simulink model "VectorCtrl_Asynchronous_VF"  (Simulink 7.9)
settings: Solver=ode23tb  StartTime=0.0  StopTime=6  RelTol=1e-3
InitFcn:
  | np=2;
  | Ts=50e-6;
  | fbase=50;
  | Vbase=440*sqrt(2/3);
libraries: powerlib x6, simulink x4, powerlib_extras x1
settings Model: Creator=H002220  LastModifiedBy=H002220

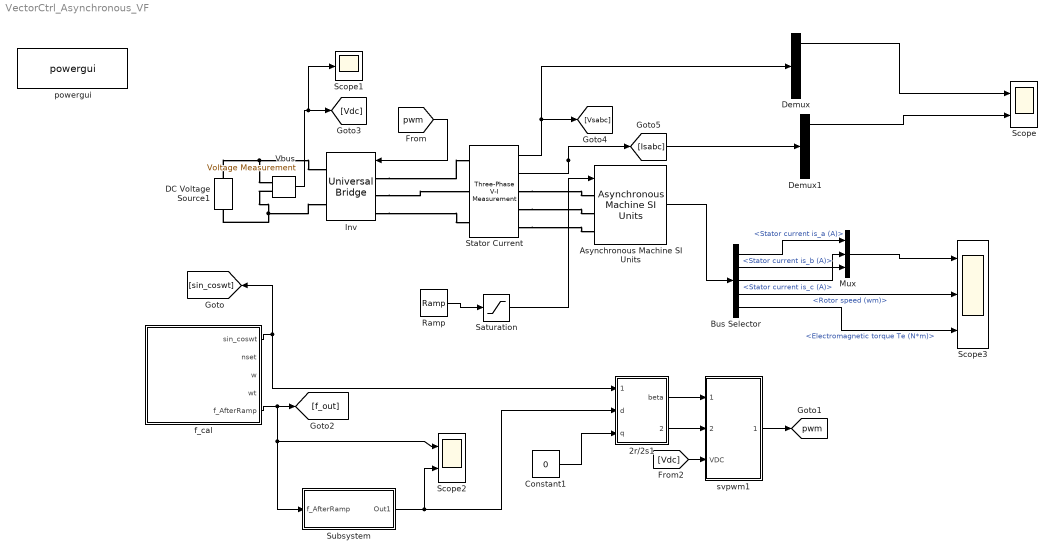
== system VectorCtrl_Asynchronous_VF ==
  2r/2s1 : Subsystem
  Asynchronous Machine SI Units : powerlib/Machines/Asynchronous Machine SI Units  PresetModel="18:  50 HP (37KW)   400 V 50Hz 1480 RPM"  MechanicalLoad=Torque Tm  ShowDetailedParameters=on  RotorType=Squirrel-cage  ReferenceFrame=Rotor  NominalParameters=[3.7e+04 400 50]  Stator=[0.08233 0.000724]  Rotor=[0.0503 0.000724]  Cage1=[ 0.022 0.226/377]  Cage2=[ 0.022 0.226/377]  Lm=0.02711  Mechanical=[0.37 0.02791 2]  PolePairs=2  InitialConditions=[1 0 0 0 0 0 0 0]  Units=SI  LoadFlowParameters=1492000  SimulateSaturation=off  Saturation=[14.03593122, 27.81365428, 53.79336849, 72.68890987, 97.98006896, 148.6815601, 215.7428561, 302.9841135, 420.4778367 ; 230, 322, 414, 460, 506, 552, 598, 644, 690]  TsPowergui=0  TsBlock=-1  IterativeModel=Forward Euler  Pmec=0
  Bus Selector : BusSelector  OutputSignals=Stator measurements.Stator current is_a (A),Stator measurements.Stator current is_b (A),Stator measurements.Stator current is_c (A),Mechanical.Rotor speed (wm),Mechanical.Electromagnetic torque Te (N*m)
  Constant1 : Constant  Value=0
  DC Voltage Source1 : powerlib/Electrical Sources/DC Voltage Source  Amplitude=600  Measurements=None
  Demux : Demux  Outputs=3
  Demux1 : Demux  Outputs=3
  Inv : powerlib/Power Electronics/Universal Bridge  Arms=3  SnubberResistance=1e5  SnubberCapacitance=inf  Device=IGBT / Diodes  Ron=1e-3  Lon=0  ForwardVoltages="[  0  0  ]"  ForwardVoltage=0  GTOparameters=[ 10e-6 , 20e-6 ]  IGBTparameters=[ 1e-6 , 2e-6 ]  Measurements=None  Measurements_2=None  converterType=Rectifier
  Mux : Mux  Inputs=3
  Ramp : simulink/Sources/Ramp  slope=4  start=0  X0=0
  Saturation : Saturate  UpperLimit=20  LowerLimit=0
  Scope : Scope  NumInputPorts=2
      settings: YMin=-5~-5  YMax=5~5  SaveName=a
  Scope1 : Scope
      settings: SaveName=ScopeData3
  Scope2 : Scope  NumInputPorts=2
      settings: YMin=-5~-5  YMax=5~5  SaveName=ScopeData4
  Scope3 : Scope  NumInputPorts=3
      settings: YMin=-5~-5~-5  YMax=5~5~5  SaveName=ScopeData5
  Stator Current : powerlib/Measurements/Three-Phase V-I Measurement  VoltageMeasurement=phase-to-phase  SetLabelV=off  LabelV=Vabc  Vpu=off  VpuLL=off  CurrentMeasurement=yes  SetLabelI=off  LabelI=Iabc  Ipu=off  Pbase=100e6  Vbase=500e3  OutputType=Complex  PhasorSimulation=off  PSBequivalent=0
  Subsystem : Subsystem
  Vbus : powerlib/Measurements/Voltage Measurement  PhasorSimulation=off  OutputType=Complex  PSBequivalent=0
  f_cal : Subsystem
  powergui : powerlib/powergui  SimulationMode=Discrete  SolverType=Tustin  SampleTime=50e-6  frequency=60  SPID=off  DisableSnubberDevices=off  DisableRonSwitches=off  DisableVfSwitches=off  SwTol=0  Interpol=off  DisplayEquations=off  FunctionMessages=off  frequencyindice=0  Pbase=100e6  ErrMax=1e-4  Iterations=50  UnitsV=kV  UnitsW=MW  echomessages=off  HookPort=off  EnableUseOfTLC=off  x0status=blocks  RestoreLinks=warning  ResistiveCurrentMeasurement=off  Frange=[0:2:500]  Ylog=off  Xlog=on  ShowGrid=off  save=off  variable=ZData  structure=a  ZoomFFT=off  StartTime=4.5  cycles=10  DisplayStyle=2  fundamental=45  FreqAxis=on  MaxFrequency=1000  frequencyindicesteady=1  RmsSteady=1  display=off  Ts=0  methode=off
  svpwm1 : Subsystem
  tag scope: pwm=global
  wires:
  2r/2s1/2(alpha) -> svpwm1/2(usaref)
  2r/2s1/1(beta) -> svpwm1/1(usbref)
  svpwm1/1(6pulse) -> [pwm]
  [Vdc] -> svpwm1/3(VDC)
  Subsystem/1(Out1) -> 2r/2s1/2(d), Scope2/2
  Constant1/1 -> 2r/2s1/3(q)
  Vbus/1 -> [Vdc], Scope1/1
  Stator Current/1 -> [Vsabc], Demux/1
  Stator Current/2 -> [Isabc], Demux1/1
  [pwm] -> Inv/1
  f_cal/5(f_AfterRamp) -> [f_out], Subsystem/1(f_AfterRamp), Scope2/1
  f_cal/1(sin_coswt) -> [sin_coswt], 2r/2s1/1(sin_cos)
  Demux/1 -> Scope/1
  Demux1/1 -> Scope/2
  Asynchronous Machine SI Units/1 -> Bus Selector/1
  Ramp/1 -> Saturation/1
  Saturation/1 -> Asynchronous Machine SI Units/1
  Bus Selector/1 -> Mux/1  "<Stator current is_a (A)>"
  Bus Selector/2 -> Mux/2  "<Stator current is_b (A)>"
  Bus Selector/3 -> Mux/3  "<Stator current is_c (A)>"
  Mux/1 -> Scope3/1
  Bus Selector/4 -> Scope3/2  "<Rotor speed (wm)>"
  Bus Selector/5 -> Scope3/3  "<Electromagnetic torque Te (N*m)>"
  connections:
  Inv/LConn1 -- Stator Current/LConn1
  Inv/LConn2 -- Stator Current/LConn2
  Inv/LConn3 -- Stator Current/LConn3
  Vbus/LConn2 -- Inv/RConn2 -- DC Voltage Source1/LConn1
  Stator Current/RConn3 -- Asynchronous Machine SI Units/LConn3
  Stator Current/RConn2 -- Asynchronous Machine SI Units/LConn2
  Stator Current/RConn1 -- Asynchronous Machine SI Units/LConn1
  DC Voltage Source1/RConn1 -- Inv/RConn1 -- Vbus/LConn1

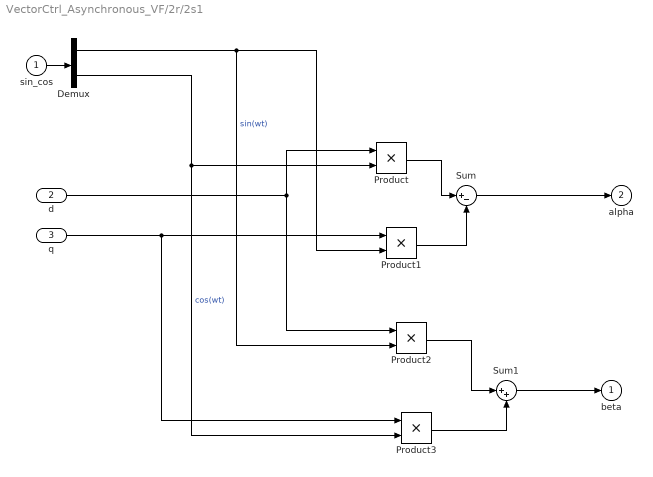
== system VectorCtrl_Asynchronous_VF/2r/2s1 ==
  sin_cos : Inport  PortDimensions=2
  d : Inport  Port=2
  q : Inport  Port=3
  Demux : Demux  Outputs=2
  Product{,1..3} (4 alike) : Product  RndMeth=Zero
  Sum : Sum  Inputs=|+-
  Sum1 : Sum  Inputs=|++
  beta : Outport  InitialOutput=0
  alpha : Outport  Port=2  InitialOutput=0
  wires:
  Sum/1 -> alpha/1
  Demux/1 -> Product1/2, Product2/2  "sin(wt)"
  Demux/2 -> Product/2, Product3/2  "cos(wt)"
  sin_cos/1 -> Demux/1
  d/1 -> Product/1, Product2/1
  q/1 -> Product1/1, Product3/1
  Product/1 -> Sum/1
  Product1/1 -> Sum/2
  Product2/1 -> Sum1/1
  Product3/1 -> Sum1/2
  Sum1/1 -> beta/1

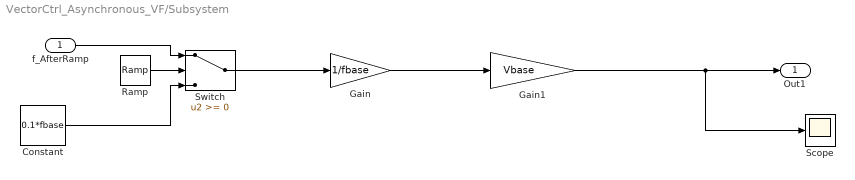
== system VectorCtrl_Asynchronous_VF/Subsystem ==
  f_AfterRamp : Inport
  Constant : Constant  Value=0.1*fbase
  Gain : Gain  Gain=1/fbase
  Gain1 : Gain  Gain=Vbase
  Ramp : simulink/Sources/Ramp  slope=1  start=0  X0=0
  Scope : Scope
      settings: SaveName=ScopeData6
  Switch : Switch
  Out1 : Outport
  wires:
  Gain/1 -> Gain1/1
  Gain1/1 -> Out1/1, Scope/1
  Ramp/1 -> Switch/2
  f_AfterRamp/1 -> Switch/1
  Constant/1 -> Switch/3
  Switch/1 -> Gain/1

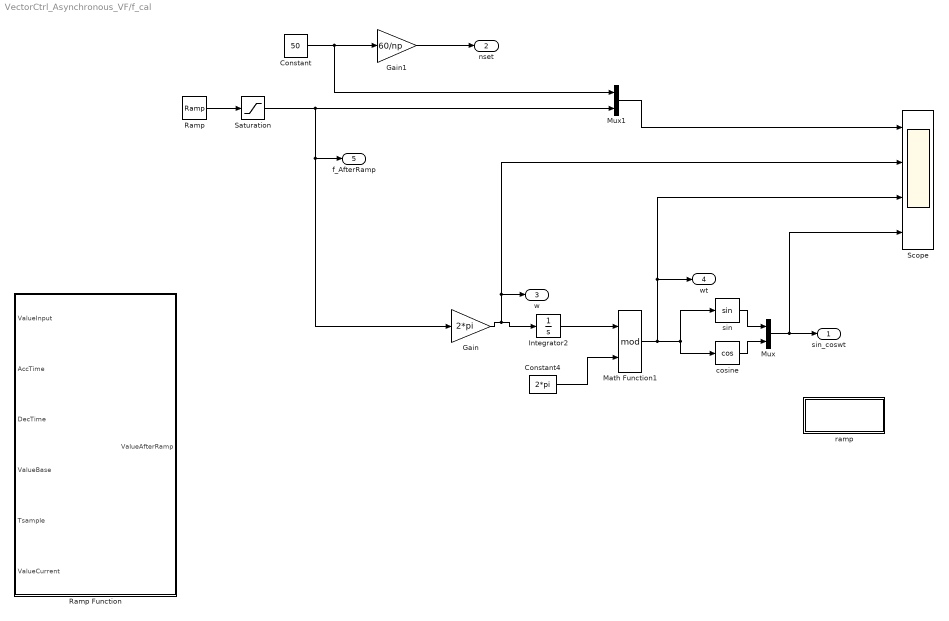
== system VectorCtrl_Asynchronous_VF/f_cal ==
  Constant : Constant  Value=50
  Constant4 : Constant  Value=2*pi
  Gain : Gain  Gain=2*pi
  Gain1 : Gain  Gain=60/np
  Integrator2 : Integrator
  Math Function1 : Math  Operator=mod  SaturateOnIntegerOverflow=on
  Mux : Mux  Inputs=2
  Mux1 : Mux  Inputs=2
  Ramp : simulink/Sources/Ramp  slope=10  start=0  X0=0
  Ramp Function : MATLAB Function  TreatAsAtomicUnit=on
  Saturation : Saturate  UpperLimit=50  LowerLimit=0
  Scope : Scope  NumInputPorts=4
      settings: YMin=-5~-5~-5~-5  YMax=5~5~5~5
  cosine : Trigonometry  Operator=cos
  ramp : Subsystem
  sin : Trigonometry
  sin_coswt : Outport
  nset : Outport  Port=2
  w : Outport  Port=3
  wt : Outport  Port=4
  f_AfterRamp : Outport  Port=5
  wires:
  sin/1 -> Mux/1
  cosine/1 -> Mux/2
  Mux/1 -> sin_coswt/1, Scope/4
  Gain1/1 -> nset/1
  Mux1/1 -> Scope/1
  Constant4/1 -> Math Function1/2
  Integrator2/1 -> Math Function1/1
  Gain/1 -> Integrator2/1, w/1, Scope/2
  Math Function1/1 -> sin/1, cosine/1, wt/1, Scope/3
  Constant/1 -> Gain1/1, Mux1/1
  Saturation/1 -> Mux1/2, f_AfterRamp/1, Gain/1
  Ramp/1 -> Saturation/1

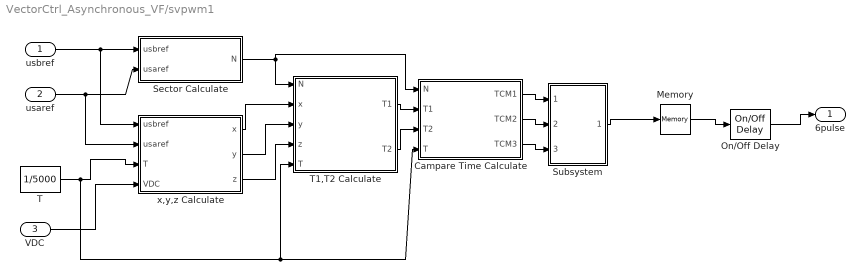
== system VectorCtrl_Asynchronous_VF/svpwm1 ==
  usbref : Inport
  usaref : Inport  Port=2
  VDC : Inport  Port=3
  Campare Time Calculate : Subsystem
  Memory : Memory
  On/Off Delay : powerlib_extras/Control  Blocks/On//Off Delay  type_delay=On delay  delay=1e-6  ic=0
  Sector Calculate : Subsystem
  Subsystem : Subsystem
  T : Constant  Value=1/5000
  T1,T2 Calculate : Subsystem
  x,y,z Calculate : Subsystem
  6pulse : Outport
  wires:
  usbref/1 -> Sector Calculate/1(usbref), x,y,z Calculate/1(usbref)
  usaref/1 -> Sector Calculate/2(usaref), x,y,z Calculate/2(usaref)
  Sector Calculate/1(N) -> T1,T2 Calculate/1(N), Campare Time Calculate/1(N)
  x,y,z Calculate/1(x) -> T1,T2 Calculate/2(x)
  x,y,z Calculate/2(y) -> T1,T2 Calculate/3(y)
  x,y,z Calculate/3(z) -> T1,T2 Calculate/4(z)
  T1,T2 Calculate/1(T1) -> Campare Time Calculate/2(T1)
  T1,T2 Calculate/2(T2) -> Campare Time Calculate/3(T2)
  Campare Time Calculate/1(TCM1) -> Subsystem/1(TCM1)
  Campare Time Calculate/2(TCM2) -> Subsystem/2(TCM2)
  Campare Time Calculate/3(TCM3) -> Subsystem/3(TCM3)
  Subsystem/1(Out1) -> Memory/1
  T/1 -> x,y,z Calculate/3(T), T1,T2 Calculate/5(T), Campare Time Calculate/4(T)
  VDC/1 -> x,y,z Calculate/4(VDC)
  Memory/1 -> On/Off Delay/1
  On/Off Delay/1 -> 6pulse/1

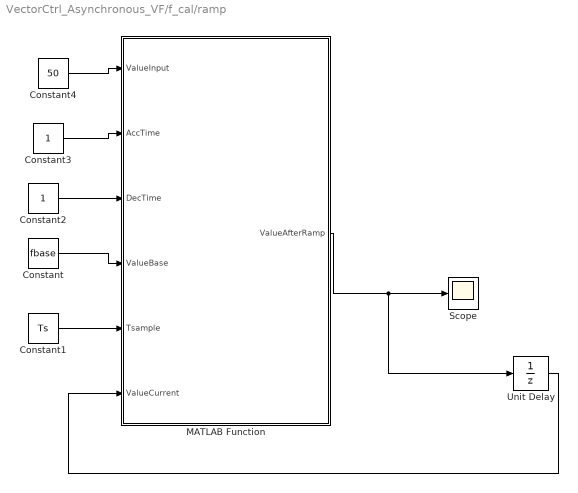
== system VectorCtrl_Asynchronous_VF/f_cal/ramp ==
  Constant : Constant  Value=fbase
  Constant1 : Constant  Value=Ts
  Constant2 : Constant
  Constant3 : Constant
  Constant4 : Constant  Value=50
  MATLAB Function : MATLAB Function  TreatAsAtomicUnit=on
  Scope : Scope
  Unit Delay : UnitDelay  SampleTime=-1
  wires:
  Constant1/1 -> MATLAB Function/5(Tsample)
  Constant/1 -> MATLAB Function/4(ValueBase)
  Constant2/1 -> MATLAB Function/3(DecTime)
  Constant3/1 -> MATLAB Function/2(AccTime)
  Constant4/1 -> MATLAB Function/1(ValueInput)
  MATLAB Function/1(ValueAfterRamp) -> Scope/1, Unit Delay/1
  Unit Delay/1 -> MATLAB Function/6(ValueCurrent)

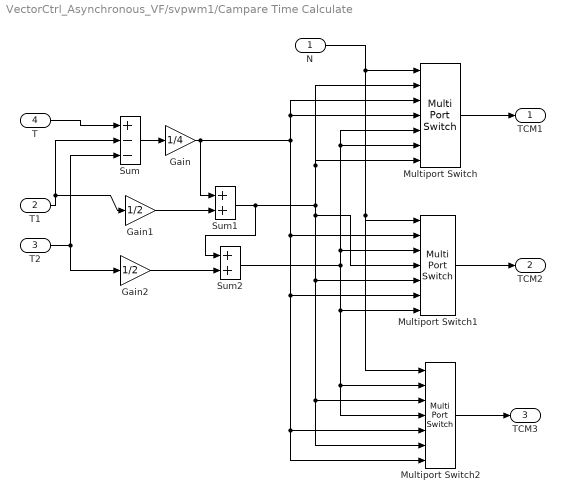
== system VectorCtrl_Asynchronous_VF/svpwm1/Campare Time Calculate ==
  N : Inport
  T1 : Inport  Port=2
  T2 : Inport  Port=3
  T : Inport  Port=4
  Gain : Gain  Gain=1/4  SaturateOnIntegerOverflow=on  OutDataTypeStr=Inherit: Same as input  ParamDataTypeStr=Inherit: Same as input
  Gain1 : Gain  Gain=1/2  SaturateOnIntegerOverflow=on  OutDataTypeStr=Inherit: Same as input  ParamDataTypeStr=Inherit: Same as input
  Gain2 : Gain  Gain=1/2  SaturateOnIntegerOverflow=on  OutDataTypeStr=Inherit: Same as input  ParamDataTypeStr=Inherit: Same as input
  Multiport Switch : MultiPortSwitch  Inputs=6  zeroidx=off  SaturateOnIntegerOverflow=on
  Multiport Switch1 : MultiPortSwitch  Inputs=6  zeroidx=off  SaturateOnIntegerOverflow=on
  Multiport Switch2 : MultiPortSwitch  Inputs=6  zeroidx=off  SaturateOnIntegerOverflow=on
  Sum : Sum  Inputs=+--  SaturateOnIntegerOverflow=on
  Sum1 : Sum  SaturateOnIntegerOverflow=on
  Sum2 : Sum  SaturateOnIntegerOverflow=on
  TCM1 : Outport
  TCM2 : Outport  Port=2
  TCM3 : Outport  Port=3
  wires:
  T/1 -> Sum/1
  T1/1 -> Sum/2, Gain1/1
  T2/1 -> Sum/3, Gain2/1
  Sum/1 -> Gain/1
  Gain/1 -> Sum1/1, Multiport Switch1/2, Multiport Switch2/5, Multiport Switch2/7, Multiport Switch1/6, Multiport Switch/3, Multiport Switch/4
  Gain1/1 -> Sum1/2
  Gain2/1 -> Sum2/2
  Multiport Switch1/1 -> TCM2/1
  Multiport Switch/1 -> TCM1/1
  Multiport Switch2/1 -> TCM3/1
  N/1 -> Multiport Switch/1, Multiport Switch2/1, Multiport Switch1/1
  Sum1/1 -> Sum2/1, Multiport Switch1/4, Multiport Switch2/3, Multiport Switch2/6, Multiport Switch1/5, Multiport Switch/2, Multiport Switch/7
  Sum2/1 -> Multiport Switch1/3, Multiport Switch/6, Multiport Switch/5, Multiport Switch2/2, Multiport Switch2/4, Multiport Switch1/7

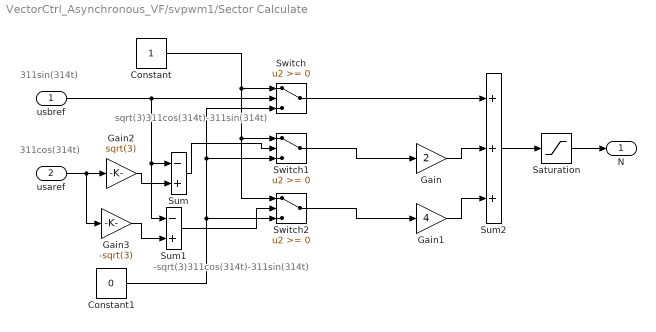
== system VectorCtrl_Asynchronous_VF/svpwm1/Sector Calculate ==
  note: 311sin(314t)
  note: 311cos(314t)
  note: sqrt(3)311cos(314t)-311sin(314t)
  note: -sqrt(3)311cos(314t)-311sin(314t)
  usbref : Inport
  usaref : Inport  Port=2
  Constant : Constant
  Constant1 : Constant  Value=0
  Gain : Gain  Gain=2  SaturateOnIntegerOverflow=on  OutDataTypeStr=Inherit: Same as input  ParamDataTypeStr=Inherit: Same as input
  Gain1 : Gain  Gain=4  SaturateOnIntegerOverflow=on  OutDataTypeStr=Inherit: Same as input  ParamDataTypeStr=Inherit: Same as input
  Gain2 : Gain  Gain=sqrt(3)  SaturateOnIntegerOverflow=on  OutDataTypeStr=Inherit: Same as input  ParamDataTypeStr=Inherit: Same as input
  Gain3 : Gain  Gain=-sqrt(3)  SaturateOnIntegerOverflow=on  OutDataTypeStr=Inherit: Same as input  ParamDataTypeStr=Inherit: Same as input
  Saturation : Saturate  UpperLimit=6  LowerLimit=1
  Sum : Sum  Inputs=-+  SaturateOnIntegerOverflow=on
  Sum1 : Sum  Inputs=-+  SaturateOnIntegerOverflow=on
  Sum2 : Sum  Inputs=+++  SaturateOnIntegerOverflow=on
  Switch : Switch  SaturateOnIntegerOverflow=on
  Switch1 : Switch  SaturateOnIntegerOverflow=on
  Switch2 : Switch  SaturateOnIntegerOverflow=on
  N : Outport
  wires:
  Constant/1 -> Switch/1, Switch1/1, Switch2/1
  usbref/1 -> Sum/1, Sum1/1, Switch/2
  Constant1/1 -> Switch/3, Switch1/3, Switch2/3
  usaref/1 -> Gain2/1, Gain3/1
  Gain2/1 -> Sum/2
  Gain3/1 -> Sum1/2
  Sum/1 -> Switch1/2
  Sum1/1 -> Switch2/2
  Switch1/1 -> Gain/1
  Switch/1 -> Sum2/1
  Gain/1 -> Sum2/2
  Gain1/1 -> Sum2/3
  Switch2/1 -> Gain1/1
  Sum2/1 -> Saturation/1
  Saturation/1 -> N/1

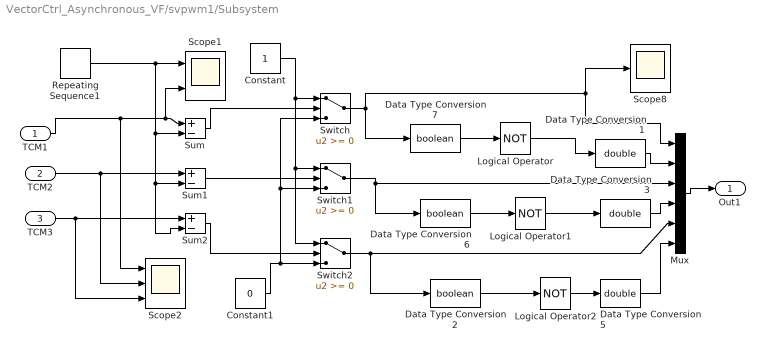
== system VectorCtrl_Asynchronous_VF/svpwm1/Subsystem ==
  TCM1 : Inport
  TCM2 : Inport  Port=2
  TCM3 : Inport  Port=3
  Constant : Constant
  Constant1 : Constant  Value=0
  Data Type Conversion1 : DataTypeConversion  OutDataTypeStr=double  SaturateOnIntegerOverflow=on  RndMeth=Zero
  Data Type Conversion2 : DataTypeConversion  OutDataTypeStr=boolean  SaturateOnIntegerOverflow=on  RndMeth=Zero
  Data Type Conversion3 : DataTypeConversion  OutDataTypeStr=double  SaturateOnIntegerOverflow=on  RndMeth=Zero
  Data Type Conversion5 : DataTypeConversion  OutDataTypeStr=double  SaturateOnIntegerOverflow=on  RndMeth=Zero
  Data Type Conversion6 : DataTypeConversion  OutDataTypeStr=boolean  SaturateOnIntegerOverflow=on  RndMeth=Zero
  Data Type Conversion7 : DataTypeConversion  OutDataTypeStr=boolean  SaturateOnIntegerOverflow=on  RndMeth=Zero
  Logical Operator : Logic  Operator=NOT  AllPortsSameDT=off
  Logical Operator1 : Logic  Operator=NOT  AllPortsSameDT=off
  Logical Operator2 : Logic  Operator=NOT  AllPortsSameDT=off
  Mux : Mux  Inputs=6
  Repeating Sequence1 : simulink/Sources/Repeating Sequence  rep_seq_t=[0 1/10000 1/5000]  rep_seq_y=[0 1/10000 0]
  Scope1 : Scope  NumInputPorts=2
      settings: TimeRange=0.028  YMin=0~2.45e-005  YMax=8.5e-005~2.64e-005  SaveName=ScopeData15
  Scope2 : Scope  NumInputPorts=3
      settings: TimeRange=0.07000000000000001  YMin=2.25e-005~2.25e-005~2.25e-005  YMax=6e-005~6e-005~6e-005  SaveName=ScopeData19
  Scope8 : Scope
      settings: TimeRange=0.07000000000000001  YMin=0  YMax=2  SaveName=ScopeData13
  Sum : Sum  Inputs=+-  SaturateOnIntegerOverflow=on
  Sum1 : Sum  Inputs=+-  SaturateOnIntegerOverflow=on
  Sum2 : Sum  Inputs=+-  SaturateOnIntegerOverflow=on
  Switch : Switch  SaturateOnIntegerOverflow=on
  Switch1 : Switch  SaturateOnIntegerOverflow=on
  Switch2 : Switch  SaturateOnIntegerOverflow=on
  Out1 : Outport
  wires:
  Constant/1 -> Switch/1, Switch1/1, Switch2/1
  Constant1/1 -> Switch2/3, Switch/3, Switch1/3
  Repeating Sequence1/1 -> Scope1/1, Sum/2, Sum2/2, Sum1/2
  TCM1/1 -> Sum/1, Scope1/2, Scope2/1
  TCM2/1 -> Sum1/1, Scope2/2
  TCM3/1 -> Sum2/1, Scope2/3
  Sum/1 -> Switch/2
  Sum1/1 -> Switch1/2
  Sum2/1 -> Switch2/2
  Mux/1 -> Out1/1
  Switch/1 -> Scope8/1, Mux/1, Data Type Conversion7/1
  Switch1/1 -> Mux/3, Data Type Conversion6/1
  Switch2/1 -> Data Type Conversion2/1, Mux/5
  Logical Operator2/1 -> Data Type Conversion5/1
  Logical Operator1/1 -> Data Type Conversion3/1
  Logical Operator/1 -> Data Type Conversion1/1
  Data Type Conversion1/1 -> Mux/2
  Data Type Conversion3/1 -> Mux/4
  Data Type Conversion5/1 -> Mux/6
  Data Type Conversion7/1 -> Logical Operator/1
  Data Type Conversion6/1 -> Logical Operator1/1
  Data Type Conversion2/1 -> Logical Operator2/1

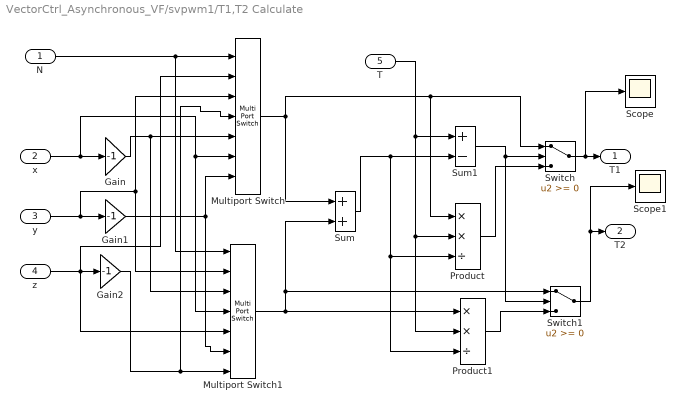
== system VectorCtrl_Asynchronous_VF/svpwm1/T1,T2 Calculate ==
  N : Inport
  x : Inport  Port=2
  y : Inport  Port=3
  z : Inport  Port=4
  T : Inport  Port=5
  Gain : Gain  Gain=-1  SaturateOnIntegerOverflow=on  OutDataTypeStr=Inherit: Same as input  ParamDataTypeStr=Inherit: Same as input
  Gain1 : Gain  Gain=-1  SaturateOnIntegerOverflow=on  OutDataTypeStr=Inherit: Same as input  ParamDataTypeStr=Inherit: Same as input
  Gain2 : Gain  Gain=-1  SaturateOnIntegerOverflow=on  OutDataTypeStr=Inherit: Same as input  ParamDataTypeStr=Inherit: Same as input
  Multiport Switch : MultiPortSwitch  Inputs=6  zeroidx=off  SaturateOnIntegerOverflow=on
  Multiport Switch1 : MultiPortSwitch  Inputs=6  zeroidx=off  SaturateOnIntegerOverflow=on
  Product : Product  Inputs=**/  SaturateOnIntegerOverflow=on  OutDataTypeStr=Inherit: Same as first input
  Product1 : Product  Inputs=**/  SaturateOnIntegerOverflow=on  OutDataTypeStr=Inherit: Same as first input
  Scope : Scope
      settings: YMin=3.5e-005  YMax=6.25e-005  SaveName=ScopeData16
  Scope1 : Scope
      settings: YMin=1.3e-007  YMax=2e-007  SaveName=ScopeData17
  Sum : Sum  SaturateOnIntegerOverflow=on
  Sum1 : Sum  Inputs=+-  SaturateOnIntegerOverflow=on
  Switch : Switch  SaturateOnIntegerOverflow=on
  Switch1 : Switch  SaturateOnIntegerOverflow=on
  T1 : Outport
  T2 : Outport  Port=2
  wires:
  N/1 -> Multiport Switch/1, Multiport Switch1/1
  x/1 -> Gain/1, Multiport Switch/6, Multiport Switch1/4
  y/1 -> Gain1/1, Multiport Switch/3, Multiport Switch1/2
  z/1 -> Gain2/1, Multiport Switch1/5, Multiport Switch/2
  Gain/1 -> Multiport Switch/5, Multiport Switch1/3
  Gain1/1 -> Multiport Switch1/6, Multiport Switch/7
  Gain2/1 -> Multiport Switch1/7, Multiport Switch/4
  Multiport Switch/1 -> Sum/1, Switch/1, Product/1
  Multiport Switch1/1 -> Product1/1, Sum/2, Switch1/1
  Switch1/1 -> T2/1, Scope1/1
  Switch/1 -> T1/1, Scope/1
  T/1 -> Sum1/1, Product1/2, Product/2
  Sum/1 -> Sum1/2, Product1/3, Product/3
  Sum1/1 -> Switch/2, Switch1/2
  Product/1 -> Switch/3
  Product1/1 -> Switch1/3

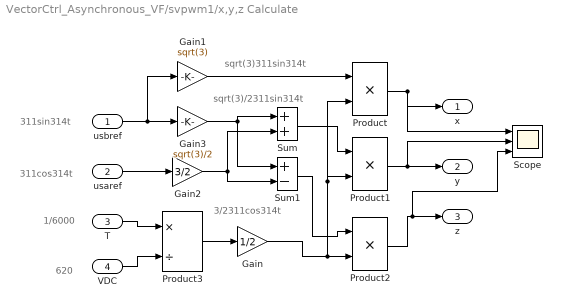
== system VectorCtrl_Asynchronous_VF/svpwm1/x,y,z Calculate ==
  note: 311sin314t
  note: 311cos314t
  note: 1/6000
  note: 620
  note: sqrt(3)311sin314t
  note: sqrt(3)/2311sin314t
  note: 3/2311cos314t
  usbref : Inport
  usaref : Inport  Port=2
  T : Inport  Port=3
  VDC : Inport  Port=4
  Gain : Gain  Gain=1/2  SaturateOnIntegerOverflow=on  OutDataTypeStr=Inherit: Same as input  ParamDataTypeStr=Inherit: Same as input
  Gain1 : Gain  Gain=sqrt(3)  SaturateOnIntegerOverflow=on  OutDataTypeStr=Inherit: Same as input  ParamDataTypeStr=Inherit: Same as input
  Gain2 : Gain  Gain=3/2  SaturateOnIntegerOverflow=on  OutDataTypeStr=Inherit: Same as input  ParamDataTypeStr=Inherit: Same as input
  Gain3 : Gain  Gain=sqrt(3)/2  SaturateOnIntegerOverflow=on  OutDataTypeStr=Inherit: Same as input  ParamDataTypeStr=Inherit: Same as input
  Product : Product  SaturateOnIntegerOverflow=on  OutDataTypeStr=Inherit: Same as first input
  Product1 : Product  SaturateOnIntegerOverflow=on  OutDataTypeStr=Inherit: Same as first input
  Product2 : Product  SaturateOnIntegerOverflow=on  OutDataTypeStr=Inherit: Same as first input
  Product3 : Product  Inputs=*/  SaturateOnIntegerOverflow=on  OutDataTypeStr=Inherit: Same as first input
  Scope : Scope  NumInputPorts=3
      settings: YMin=-8e-005~-8e-005~-8e-005  YMax=8e-005~8e-005~8e-005  SaveName=ScopeData18
  Sum : Sum  SaturateOnIntegerOverflow=on
  Sum1 : Sum  Inputs=+-  SaturateOnIntegerOverflow=on
  x : Outport
  y : Outport  Port=2
  z : Outport  Port=3
  wires:
  T/1 -> Product3/1
  VDC/1 -> Product3/2
  usaref/1 -> Gain2/1
  usbref/1 -> Gain3/1, Gain1/1
  Gain1/1 -> Product/1
  Gain/1 -> Product2/2, Product1/2, Product/2
  Gain3/1 -> Sum/1, Sum1/1
  Gain2/1 -> Sum1/2, Sum/2
  Sum/1 -> Product1/1
  Sum1/1 -> Product2/1
  Product/1 -> x/1, Scope/1
  Product1/1 -> y/1, Scope/2
  Product2/1 -> z/1, Scope/3
  Product3/1 -> Gain/1

== matlab function f_cal/Ramp Function ==
  data: ValueInput input double; ValueAfterRamp output double; AccTime input double; DecTime input double; ValueBase input double; Tsample input double; ValueCurrent input double
function ValueAfterRamp = fcn(ValueInput,AccTime,DecTime,ValueBase, Tsample, ValueCurrent)
%#codegen
%syms ValueCurrent;
%persistent ValueCurrent;
StepAcc = ValueBase*Tsample/AccTime;
StepDec = ValueBase*Tsample/DecTime;
if ValueInput > ValueCurrent;
    if (ValueInput - ValueCurrent)<StepAcc;
        ValueAfterRamp = ValueInput;
    else 
        ValueAfterRamp = ValueCurrent + StepAcc;
    end
elseif ValueInput < ValueCurrent;
    if (ValueCurrent - ValueInput)<StepDec;
        ValueAfterRamp = ValueInput;
    else 
        ValueAfterRamp = ValueCurrent - StepDec;
    end
else 
    ValueAfterRamp = ValueInput;
end
%ValueCurrent = ValueAfterRamp;
%ValueAfterRamp = ValueInput;

== matlab function f_cal/ramp/MATLAB Function ==
  data: ValueInput input double; ValueAfterRamp output double; AccTime input double; DecTime input double; ValueBase input double; Tsample input double; ValueCurrent input double
function ValueAfterRamp = fcn(ValueInput,AccTime,DecTime,ValueBase, Tsample, ValueCurrent)
%#codegen
%syms ValueCurrent;
%persistent ValueCurrent;
StepAcc = ValueBase*Tsample/AccTime;
StepDec = ValueBase*Tsample/DecTime;
if ValueInput > ValueCurrent;
    if (ValueInput - ValueCurrent)<StepAcc;
        ValueAfterRamp = ValueInput;
    else 
        ValueAfterRamp = ValueCurrent + StepAcc;
    end
elseif ValueInput < ValueCurrent;
    if (ValueCurrent - ValueInput)<StepDec;
        ValueAfterRamp = ValueInput;
    else 
        ValueAfterRamp = ValueCurrent - StepDec;
    end
else 
    ValueAfterRamp = ValueInput;
end
%ValueCurrent = ValueAfterRamp;
%ValueAfterRamp = ValueInput;
